simulink model "rtwdemo_logicORsf"  (Simulink 7.1)
settings: Solver=FixedStepDiscrete  StartTime=0.0  StopTime=10.0  RelTol=1e-3
settings Model: Creator=ajayaram  LastModifiedBy=ajayaram
settings OptimizationCC: OptimizeModelRefInitCode=on  LifeSpan=1
settings RTWCC: SystemTargetFile=ert.tlc  GenCodeOnly=on  GenerateMakefile=off  TemplateMakefile=ert_default_tmf  Description=Real-Time Workshop Embedded Coder (no auto configuration)  GenerateReport=on  ProcessScript=ert_make_rtw_hook  IncludeHyperlinkInReport=on  LaunchReport=on
settings CodeAppCC: GenerateComments=off  IgnoreCustomStorageClasses=off  SimulinkBlockComments=off
settings ERTTargetCC: GenerateSampleERTMain=on  InlinedParameterPlacement=NonHierarchical  ERTCustomFileTemplate=example_file_process.tlc

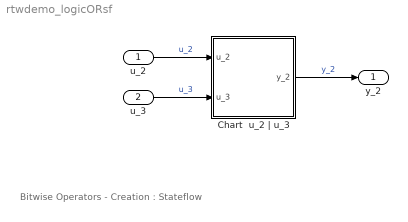
== system rtwdemo_logicORsf ==
  note: Bitwise Operators - Creation : Stateflow
  u_2 : Inport  DataType=uint8  OutDataType=sfix(16)  OutScaling=2^0  OutDataTypeStr=uint8
  u_3 : Inport  Port=2  DataType=uint8  OutDataType=sfix(16)  OutScaling=2^0  OutDataTypeStr=uint8
  Chart  u_2 | u_3 : Stateflow chart
  y_2 : Outport  OutDataType=sfix(16)  OutScaling=2^0
  wires:
  Chart  u_2 | u_3/1(y_2) -> y_2/1  "y_2"
  u_2/1 -> Chart  u_2 | u_3/1(u_2)  "u_2"
  u_3/1 -> Chart  u_2 | u_3/2(u_3)  "u_3"

== stateflow chart Chart u_2 | u_3 ==
  (junction 4) -> (junction 3) : {
      |   y_2 = u_2 | u_3 ;
      | }
  (default) -> (junction 4)
  data: u_2 input uint8; u_3 input uint8; y_2 output uint8
